simulink library "satelliteDynamics_lib_old"  (R2018b)
settings: Solver=ode45  StartTime=0.0  StopTime=10.0  RelTol=1e-3  EnableMultiTasking=on
undefined symbols (not defined in the file): DiscIntNeverNeededParam, fswParams, simParams
libraries: vrlib x1, aerolibutil x1
settings Model: Creator=devantormey  LastModifiedBy=colem
settings DataIOCC: LimitDataPoints=on
settings OptimizationCC: LifeSpan=inf
settings DebuggingCC: AllowSymbolicDim=off  SFUnexpectedBacktrackingDiag=warning  SFNoUnconditionalDefaultTransitionDiag=warning
settings SFSimCC: SimUseLocalCustomCode=off
settings RTWCC: RTWUseLocalCustomCode=off
settings CodeAppCC: StateflowObjectComments=on
settings GRTTargetCC: TargetLangStandard=C89/C90 (ANSI)  GeneratePreprocessorConditionals=Disable all
settings ConfigComp: CovMetricSettings=dw  CovHtmlReporting=on  CovSaveCumulativeToWorkspaceVar=on  CovSaveSingleToWorkspaceVar=on  CovExternalEMLEnable=off

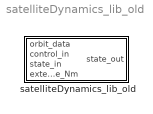
== system satelliteDynamics_lib_old ==
  satelliteDynamics_lib_old : Subsystem

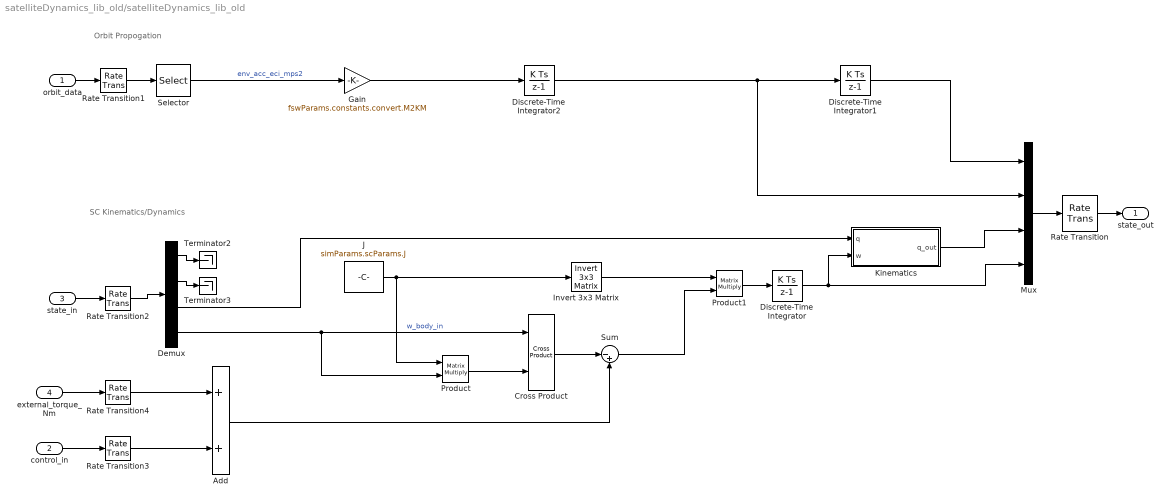
== system satelliteDynamics_lib_old/satelliteDynamics_lib_old ==
  note: Orbit Propogation
  note: SC Kinematics/Dynamics
  orbit_data : Inport
  control_in : Inport  Port=2
  state_in : Inport  Port=3
  external_torque_Nm : Inport  Port=4
  Add : Sum
  Cross Product : vrlib/Utilities/Cross Product
      settings: SourceProductBaseCode=VR
  Demux : Demux  Outputs=[3 3 4 3]
  Discrete-Time Integrator : DiscreteIntegrator  InitialCondition=simParams.initialConditions.w0  SampleTime=-1  ICPrevOutput=DiscIntNeverNeededParam  ICPrevScaledInput=DiscIntNeverNeededParam
  Discrete-Time Integrator1 : DiscreteIntegrator  InitialCondition=simParams.initialConditions.r0  SampleTime=-1  ICPrevOutput=DiscIntNeverNeededParam  ICPrevScaledInput=DiscIntNeverNeededParam
  Discrete-Time Integrator2 : DiscreteIntegrator  InitialCondition=simParams.initialConditions.v0  SampleTime=-1  ICPrevOutput=DiscIntNeverNeededParam  ICPrevScaledInput=DiscIntNeverNeededParam
  Gain : Gain  Gain=fswParams.constants.convert.M2KM
  Invert 3x3 Matrix : aerolibutil/Invert  3x3 Matrix
  J : Constant  Value=simParams.scParams.J
  Kinematics : Subsystem
  Mux : Mux  Inputs=[3 3 4 3]
  Product : Product  Multiplication=Matrix(*)
  Product1 : Product  Multiplication=Matrix(*)
  Rate Transition : RateTransition  InitialCondition=[simParams.initialConditions.r0;simParams.initialConditions.v0;simParams.initialConditions.q0;simParams.initialConditions.w0]
  Rate Transition1 : RateTransition  OutPortSampleTime=simParams.sample_time_s
  Rate Transition2 : RateTransition  InitialCondition=[simParams.initialConditions.r0;simParams.initialConditions.v0;simParams.initialConditions.q0;simParams.initialConditions.w0]  OutPortSampleTime=simParams.sample_time_s
  Rate Transition3 : RateTransition  OutPortSampleTime=simParams.sample_time_s
  Rate Transition4 : RateTransition  OutPortSampleTime=simParams.sample_time_s
  Selector : Selector  InputPortWidth=13  IndexOptions=Index vector (dialog)  Indices=[1 2 3]  OutputSizes=1
  Sum : Sum  Inputs=|-+
  Terminator2 : Terminator
  Terminator3 : Terminator
  state_out : Outport
  wires:
  J/1 -> Product/1, Invert 3x3 Matrix/1
  Product/1 -> Cross Product/2
  control_in/1 -> Rate Transition3/1
  Cross Product/1 -> Sum/1
  Sum/1 -> Product1/2
  Invert 3x3 Matrix/1 -> Product1/1
  Product1/1 -> Discrete-Time Integrator/1
  Discrete-Time Integrator/1 -> Mux/4, Kinematics/2(w)
  Kinematics/1(q_out) -> Mux/3
  Mux/1 -> Rate Transition/1
  Demux/4 -> Cross Product/1, Product/2  "w_body_in"
  Discrete-Time Integrator2/1 -> Mux/2, Discrete-Time Integrator1/1
  Discrete-Time Integrator1/1 -> Mux/1
  Gain/1 -> Discrete-Time Integrator2/1
  Demux/3 -> Kinematics/1(q)
  Demux/1 -> Terminator2/1
  Rate Transition/1 -> state_out/1
  orbit_data/1 -> Rate Transition1/1
  Rate Transition1/1 -> Selector/1
  state_in/1 -> Rate Transition2/1
  Rate Transition2/1 -> Demux/1
  external_torque_Nm/1 -> Rate Transition4/1
  Rate Transition4/1 -> Add/1
  Rate Transition3/1 -> Add/2
  Add/1 -> Sum/2
  Demux/2 -> Terminator3/1
  Selector/1 -> Gain/1  "env_acc_eci_mps2"

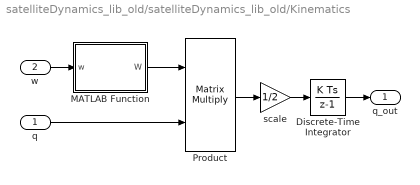
== system satelliteDynamics_lib_old/satelliteDynamics_lib_old/Kinematics ==
  q : Inport
  w : Inport  Port=2
  Discrete-Time Integrator : DiscreteIntegrator  InitialCondition=simParams.initialConditions.q0  SampleTime=-1  ICPrevOutput=DiscIntNeverNeededParam  ICPrevScaledInput=DiscIntNeverNeededParam
  MATLAB Function : MATLAB Function  TreatAsAtomicUnit=on
  Product : Product  Multiplication=Matrix(*)
  scale : Gain  Gain=1/2
  q_out : Outport
  wires:
  w/1 -> MATLAB Function/1(w)
  MATLAB Function/1(W) -> Product/1
  q/1 -> Product/2
  Product/1 -> scale/1
  scale/1 -> Discrete-Time Integrator/1
  Discrete-Time Integrator/1 -> q_out/1

== matlab function satelliteDynamics_lib_old/Kinematics/MATLAB Function ==
  data: w input; W output
function W = fcn(w)
%#codegen

W = [0, -w(1),-w(2),-w(3); w(1), 0,w(3), -w(2); w(2), -w(3), 0, w(1); w(3), w(2), -w(1), 0 ];

end
